simulink model "graph2"  (R2019a)
settings: Solver=VariableStepAuto  StartTime=0.0  StopTime=10.0  RelTol=1e-3
undefined symbols (not defined in the file or in its folder): av_simple, car, car_acc, genericAgentLib, LargeScaleSimLib_old, Objects, X, Y
libraries: robotlib x28, simulink x2
settings Model: Creator=agc3  LastModifiedBy=agc3

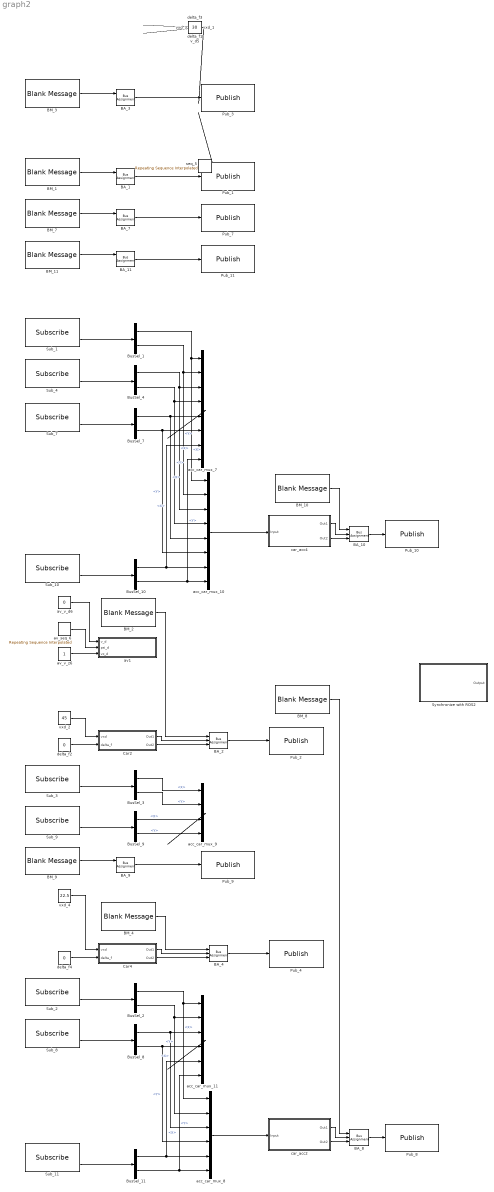
== system graph2 ==
  BA_{1..4,7..11} (9 alike) : BusAssignment  AssignedSignals=X,Y
  BM_{1..4,7..11} (9 alike) : robotlib/Blank Message  messageClass=Message  entityType=geometry_msgs/Point  messageType=geometry_msgs/Point  SampleTime=inf
      settings: SourceProductBaseCode=RO
  BusSel_{1..4,7..11} (9 alike) : BusSelector  OutputSignals=X,Y
  Car2 : Subsystem  AncestorBlock=LargeScaleSimLib_old/car  mask{obj=Objects{2}}
      mask prompts: obj "object"
      mask init:
      | set_param([gcb,'/ToWS'],'VariableName',obj.NameStrh)
  Car4 : Subsystem  AncestorBlock=LargeScaleSimLib_old/car  mask{obj=Objects{4}}
      mask prompts: obj "object"
      mask init:
      | set_param([gcb,'/ToWS'],'VariableName',obj.NameStrh)
  Pub_1 : robotlib/Publish  topicSource=Select from ROS network  topic=/Data_Pub_1  messageType=geometry_msgs/Point  messageQueueLength=1
      settings: SourceProductBaseCode=RO
  Pub_10 : robotlib/Publish  topicSource=Select from ROS network  topic=/Data_Pub_10  messageType=geometry_msgs/Point  messageQueueLength=1
      settings: SourceProductBaseCode=RO
  Pub_11 : robotlib/Publish  topicSource=Select from ROS network  topic=/Data_Pub_11  messageType=geometry_msgs/Point  messageQueueLength=1
      settings: SourceProductBaseCode=RO
  Pub_2 : robotlib/Publish  topicSource=Select from ROS network  topic=/Data_Pub_2  messageType=geometry_msgs/Point  messageQueueLength=1
      settings: SourceProductBaseCode=RO
  Pub_3 : robotlib/Publish  topicSource=Select from ROS network  topic=/Data_Pub_3  messageType=geometry_msgs/Point  messageQueueLength=1
      settings: SourceProductBaseCode=RO
  Pub_4 : robotlib/Publish  topicSource=Select from ROS network  topic=/Data_Pub_4  messageType=geometry_msgs/Point  messageQueueLength=1
      settings: SourceProductBaseCode=RO
  Pub_7 : robotlib/Publish  topicSource=Select from ROS network  topic=/Data_Pub_7  messageType=geometry_msgs/Point  messageQueueLength=1
      settings: SourceProductBaseCode=RO
  Pub_8 : robotlib/Publish  topicSource=Select from ROS network  topic=/Data_Pub_8  messageType=geometry_msgs/Point  messageQueueLength=1
      settings: SourceProductBaseCode=RO
  Pub_9 : robotlib/Publish  topicSource=Select from ROS network  topic=/Data_Pub_9  messageType=geometry_msgs/Point  messageQueueLength=1
      settings: SourceProductBaseCode=RO
  Sub_1 : robotlib/Subscribe  topicSource=Select from ROS network  topic=/Data_Pub_1  messageType=geometry_msgs/Point  sampleTime=-1  messageQueueLength=1
      settings: SourceProductBaseCode=RO
  Sub_10 : robotlib/Subscribe  topicSource=Select from ROS network  topic=/Data_Pub_10  messageType=geometry_msgs/Point  sampleTime=-1  messageQueueLength=1
      settings: SourceProductBaseCode=RO
  Sub_11 : robotlib/Subscribe  topicSource=Select from ROS network  topic=/Data_Pub_11  messageType=geometry_msgs/Point  sampleTime=-1  messageQueueLength=1
      settings: SourceProductBaseCode=RO
  Sub_2 : robotlib/Subscribe  topicSource=Select from ROS network  topic=/Data_Pub_2  messageType=geometry_msgs/Point  sampleTime=-1  messageQueueLength=1
      settings: SourceProductBaseCode=RO
  Sub_3 : robotlib/Subscribe  topicSource=Select from ROS network  topic=/Data_Pub_3  messageType=geometry_msgs/Point  sampleTime=-1  messageQueueLength=1
      settings: SourceProductBaseCode=RO
  Sub_4 : robotlib/Subscribe  topicSource=Select from ROS network  topic=/Data_Pub_4  messageType=geometry_msgs/Point  sampleTime=-1  messageQueueLength=1
      settings: SourceProductBaseCode=RO
  Sub_7 : robotlib/Subscribe  topicSource=Select from ROS network  topic=/Data_Pub_7  messageType=geometry_msgs/Point  sampleTime=-1  messageQueueLength=1
      settings: SourceProductBaseCode=RO
  Sub_8 : robotlib/Subscribe  topicSource=Select from ROS network  topic=/Data_Pub_8  messageType=geometry_msgs/Point  sampleTime=-1  messageQueueLength=1
      settings: SourceProductBaseCode=RO
  Sub_9 : robotlib/Subscribe  topicSource=Select from ROS network  topic=/Data_Pub_9  messageType=geometry_msgs/Point  sampleTime=-1  messageQueueLength=1
      settings: SourceProductBaseCode=RO
  Synchronize with ROS2 : Subsystem  Priority=1  TreatAsAtomicUnit=on
  acc_car_mux_10 : Mux  Inputs=8
  acc_car_mux_11 : Mux  Inputs=6
  acc_car_mux_7 : Mux  Inputs=8
  acc_car_mux_8 : Mux  Inputs=6
  acc_car_mux_9 : Mux
  av1 : Subsystem  AncestorBlock=genericAgentLib/av_simple  mask{obj=Objects{6}}
      mask prompts: obj "object"
      mask init:
      | set_param([gcb,'/ToWS'],'VariableName',obj.NameStrh)
  av_seq_6 : simulink/Sources/Repeating Sequence Interpolated  OutValues=[3 1 4 2 1].'  TimeValues=[0 0.1 0.5 0.6 1].'  LookUpMeth=Interpolation-Use End Values  tsamp=-1  OutMin=[]  OutMax=[]  OutDataTypeStr=double  OutputDataTypeScalingMode=double  OutDataType=fixdt(0,8)  OutScaling=2^-10
  av_v_d6 : Constant  Value=0
  av_v_z6 : Constant
  car_acc2 : Subsystem  AncestorBlock=LargeScaleSimLib_old/car_acc  mask{obj=Objects{8}}
      mask prompts: obj "object"
  car_acc4 : Subsystem  AncestorBlock=LargeScaleSimLib_old/car_acc  mask{obj=Objects{10}}
      mask prompts: obj "object"
  delta_f{1..4} (4 alike) : Constant  Value=0
  seq_5 : simulink/Sources/Repeating Sequence Interpolated  OutValues=[3 1 4 2 1].'  TimeValues=[0 0.1 0.5 0.6 1].'  LookUpMeth=Interpolation-Use End Values  tsamp=-1  OutMin=[]  OutMax=[]  OutDataTypeStr=double  OutputDataTypeScalingMode=double  OutDataType=fixdt(0,8)  OutScaling=2^-10
  v_d5 : Constant  Value=7.4003
  vxd_1 : Constant  Value=90
  vxd_2 : Constant  Value=45
  vxd_3 : Constant  Value=30
  vxd_4 : Constant  Value=22.5
  wires:
  ? -> BA_1/2
  ? -> BA_1/3
  vxd_1/1 -> ?
  delta_f1/1 -> ?
  ? -> BA_3/2
  ? -> BA_3/3
  vxd_3/1 -> ?
  delta_f3/1 -> ?
  v_d5/1 -> ?
  seq_5/1 -> ?
  ? -> BA_7/2
  ? -> BA_7/3
  acc_car_mux_7/1 -> ?
  ? -> BA_9/2
  ? -> BA_9/3
  acc_car_mux_9/1 -> ?
  ? -> BA_11/2
  ? -> BA_11/3
  acc_car_mux_11/1 -> ?
  BusSel_1/1 -> acc_car_mux_7/1, acc_car_mux_10/1  "<X>"
  BusSel_4/1 -> acc_car_mux_7/3, acc_car_mux_10/3  "<X>"
  BusSel_7/1 -> acc_car_mux_7/5, acc_car_mux_10/5  "<X>"
  BusSel_4/2 -> acc_car_mux_7/4, acc_car_mux_10/4  "<Y>"
  BusSel_10/2 -> acc_car_mux_7/8, acc_car_mux_10/8  "<Y>"
  BusSel_8/2 -> acc_car_mux_8/4, acc_car_mux_11/4  "<Y>"
  BusSel_11/2 -> acc_car_mux_8/6, acc_car_mux_11/6  "<Y>"
  BA_1/1 -> Pub_1/1
  BM_10/1 -> BA_10/1
  BusSel_10/1 -> acc_car_mux_7/7, acc_car_mux_10/7  "<X>"
  car_acc4/1(Out1) -> BA_10/2
  Car4/2(Out2) -> BA_4/3
  BusSel_9/1 -> acc_car_mux_9/3  "<X>"
  BM_2/1 -> BA_2/1
  car_acc4/2(Out2) -> BA_10/3
  BM_9/1 -> BA_9/1
  BA_10/1 -> Pub_10/1
  BM_11/1 -> BA_11/1
  Sub_8/2 -> BusSel_8/1
  Sub_3/2 -> BusSel_3/1
  BA_8/1 -> Pub_8/1
  BusSel_8/1 -> acc_car_mux_8/3, acc_car_mux_11/3  "<X>"
  Car4/1(Out1) -> BA_4/2
  BA_11/1 -> Pub_11/1
  BusSel_2/1 -> acc_car_mux_8/1, acc_car_mux_11/1  "<X>"
  BA_2/1 -> Pub_2/1
  BusSel_7/2 -> acc_car_mux_7/6, acc_car_mux_10/6  "<Y>"
  BusSel_3/1 -> acc_car_mux_9/1  "<X>"
  acc_car_mux_10/1 -> car_acc4/1(Input)
  BusSel_11/1 -> acc_car_mux_8/5, acc_car_mux_11/5  "<X>"
  BM_7/1 -> BA_7/1
  Sub_9/2 -> BusSel_9/1
  BusSel_3/2 -> acc_car_mux_9/2  "<Y>"
  acc_car_mux_8/1 -> car_acc2/1(Input)
  car_acc2/2(Out2) -> BA_8/3
  BM_8/1 -> BA_8/1
  BusSel_9/2 -> acc_car_mux_9/4  "<Y>"
  Sub_7/2 -> BusSel_7/1
  Car2/1(Out1) -> BA_2/2
  Sub_10/2 -> BusSel_10/1
  BusSel_2/2 -> acc_car_mux_8/2, acc_car_mux_11/2  "<Y>"
  Sub_4/2 -> BusSel_4/1
  Sub_1/2 -> BusSel_1/1
  car_acc2/1(Out1) -> BA_8/2
  BA_7/1 -> Pub_7/1
  Car2/2(Out2) -> BA_2/3
  delta_f4/1 -> Car4/2(delta_f)
  av_seq_6/1 -> av1/2(psi_d)
  av_v_d6/1 -> av1/1(v_d)
  Sub_11/2 -> BusSel_11/1
  vxd_4/1 -> Car4/1("vxd ")
  BM_1/1 -> BA_1/1
  vxd_2/1 -> Car2/1("vxd ")
  BA_9/1 -> Pub_9/1
  BA_4/1 -> Pub_4/1
  BusSel_1/2 -> acc_car_mux_7/2, acc_car_mux_10/2  "<Y>"
  BM_4/1 -> BA_4/1
  Sub_2/2 -> BusSel_2/1
  BA_3/1 -> Pub_3/1
  av_v_z6/1 -> av1/3(vz_d)
  BM_3/1 -> BA_3/1
  delta_f2/1 -> Car2/2(delta_f)

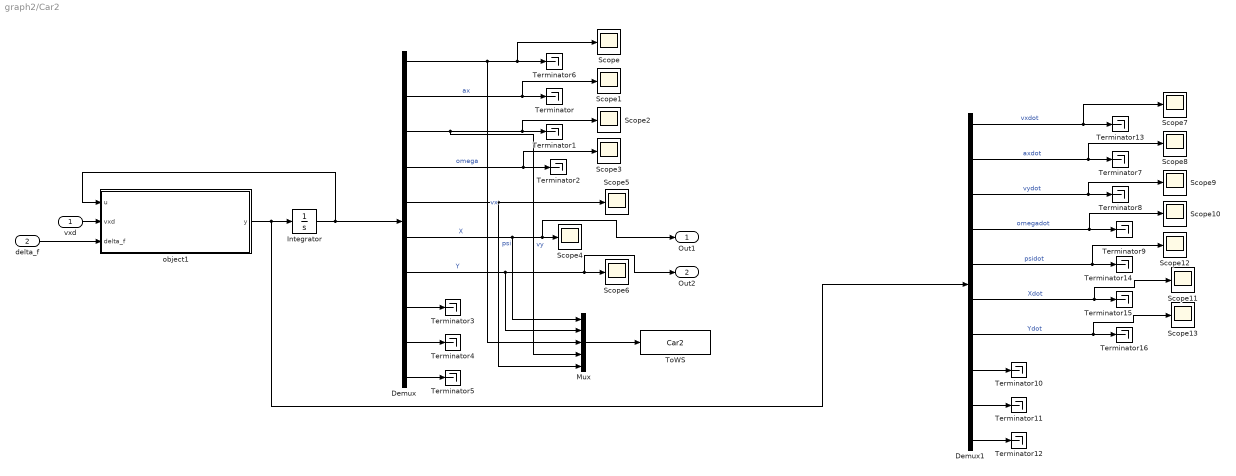
== system graph2/Car2 ==
  "vxd " : Inport
  delta_f : Inport  Port=2
  Demux : Demux  Outputs=10
  Demux1 : Demux  Outputs=10
  Integrator : Integrator  InitialCondition=obj.init
  Mux : Mux  Inputs=5
  Scope{,1..13} (14 alike) : Scope
  Terminator{,1..16} (17 alike) : Terminator
  ToWS : ToWorkspace  VariableName=Car2  SaveFormat=Timeseries  SampleTime=-1
  object1 : MATLAB Function  TreatAsAtomicUnit=on
  Out1 : Outport  VectorParamsAs1DForOutWhenUnconnected=on
  Out2 : Outport  Port=2  VectorParamsAs1DForOutWhenUnconnected=on
  wires:
  "vxd "/1 -> object1/2(vxd)
  Mux/1 -> ToWS/1
  object1/1(y) -> Integrator/1, Demux1/1
  Demux1/1 -> Scope7/1, Terminator13/1  "vxdot"
  Demux1/2 -> Scope8/1, Terminator7/1  "axdot"
  Demux1/3 -> Scope9/1, Terminator8/1  "vydot"
  Demux1/4 -> Scope10/1, Terminator9/1  "omegadot"
  Demux1/5 -> Scope12/1, Terminator14/1  "psidot"
  Demux1/6 -> Scope11/1, Terminator15/1  "Xdot"
  Demux1/7 -> Scope13/1, Terminator16/1  "Ydot"
  Demux1/8 -> Terminator10/1
  Demux1/9 -> Terminator11/1
  Demux1/10 -> Terminator12/1
  Demux/10 -> Terminator5/1
  Demux/9 -> Terminator4/1
  Demux/8 -> Terminator3/1
  Demux/7 -> Scope6/1, Out2/1, Mux/2  "Y"
  Demux/6 -> Scope4/1, Out1/1, Mux/1  "X"
  Demux/5 -> Scope5/1, Mux/5  "psi"
  Demux/4 -> Terminator2/1, Scope3/1  "omega"
  Demux/3 -> Terminator1/1, Scope2/1, Mux/4  "vy"
  Demux/2 -> Terminator/1, Scope1/1  "ax"
  Demux/1 -> Terminator6/1, Scope/1, Mux/3  "vx"
  delta_f/1 -> object1/3(delta_f)
  Integrator/1 -> object1/1(u), Demux/1

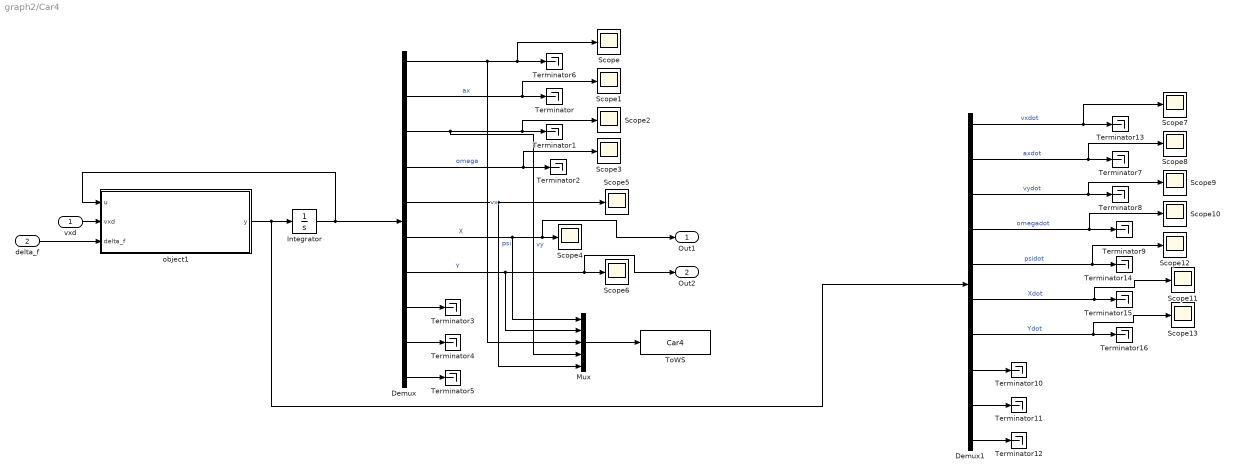
== system graph2/Car4 ==
  "vxd " : Inport
  delta_f : Inport  Port=2
  Demux : Demux  Outputs=10
  Demux1 : Demux  Outputs=10
  Integrator : Integrator  InitialCondition=obj.init
  Mux : Mux  Inputs=5
  Scope{,1..13} (14 alike) : Scope
  Terminator{,1..16} (17 alike) : Terminator
  ToWS : ToWorkspace  VariableName=Car4  SaveFormat=Timeseries  SampleTime=-1
  object1 : MATLAB Function  TreatAsAtomicUnit=on
  Out1 : Outport  VectorParamsAs1DForOutWhenUnconnected=on
  Out2 : Outport  Port=2  VectorParamsAs1DForOutWhenUnconnected=on
  wires:
  "vxd "/1 -> object1/2(vxd)
  Mux/1 -> ToWS/1
  object1/1(y) -> Integrator/1, Demux1/1
  Demux1/1 -> Scope7/1, Terminator13/1  "vxdot"
  Demux1/2 -> Scope8/1, Terminator7/1  "axdot"
  Demux1/3 -> Scope9/1, Terminator8/1  "vydot"
  Demux1/4 -> Scope10/1, Terminator9/1  "omegadot"
  Demux1/5 -> Scope12/1, Terminator14/1  "psidot"
  Demux1/6 -> Scope11/1, Terminator15/1  "Xdot"
  Demux1/7 -> Scope13/1, Terminator16/1  "Ydot"
  Demux1/8 -> Terminator10/1
  Demux1/9 -> Terminator11/1
  Demux1/10 -> Terminator12/1
  Demux/10 -> Terminator5/1
  Demux/9 -> Terminator4/1
  Demux/8 -> Terminator3/1
  Demux/7 -> Scope6/1, Out2/1, Mux/2  "Y"
  Demux/6 -> Scope4/1, Out1/1, Mux/1  "X"
  Demux/5 -> Scope5/1, Mux/5  "psi"
  Demux/4 -> Terminator2/1, Scope3/1  "omega"
  Demux/3 -> Terminator1/1, Scope2/1, Mux/4  "vy"
  Demux/2 -> Terminator/1, Scope1/1  "ax"
  Demux/1 -> Terminator6/1, Scope/1, Mux/3  "vx"
  delta_f/1 -> object1/3(delta_f)
  Integrator/1 -> object1/1(u), Demux/1

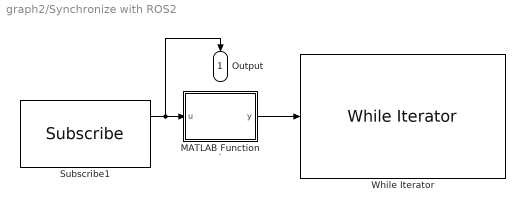
== system graph2/Synchronize with ROS2 ==
  note: `
  MATLAB Function : MATLAB Function  TreatAsAtomicUnit=on
  Subscribe1 : robotlib/Subscribe  topicSource=Select from ROS network  topic=/ClockTick  messageType=std_msgs/Float64  sampleTime=-1  messageQueueLength=1
      settings: SourceProductBaseCode=RO
  While Iterator : WhileIterator  MaxIters=-1  WhileBlockType=do-while  ShowIterationPort=on
  Output : Outport
  wires:
  Subscribe1/1 -> Output/1, MATLAB Function/1(u)
  MATLAB Function/1(y) -> While Iterator/1

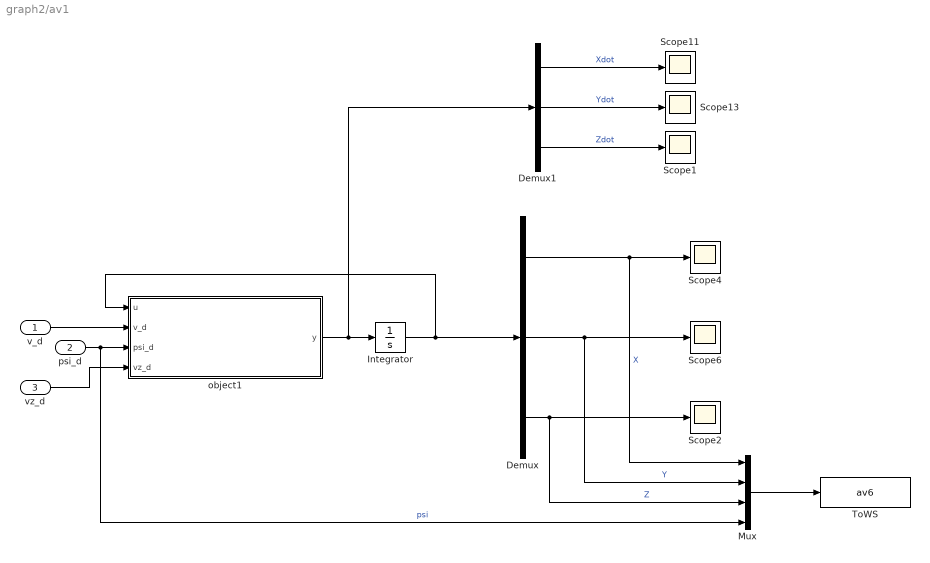
== system graph2/av1 ==
  v_d : Inport
  psi_d : Inport  Port=2
  vz_d : Inport  Port=3
  Demux : Demux  Outputs=3
  Demux1 : Demux  Outputs=3
  Integrator : Integrator  InitialCondition=obj.init
  Mux : Mux
  Scope{1..2,4,6,11,13} (6 alike) : Scope
  ToWS : ToWorkspace  VariableName=av6  SaveFormat=Timeseries  SampleTime=-1
  object1 : MATLAB Function  TreatAsAtomicUnit=on
  wires:
  Demux/2 -> Mux/2, Scope6/1  "Y"
  Demux/1 -> Mux/1, Scope4/1  "X"
  psi_d/1 -> Mux/4, object1/3(psi_d)  "psi"
  v_d/1 -> object1/2(v_d)
  Mux/1 -> ToWS/1
  object1/1(y) -> Integrator/1, Demux1/1
  Demux1/1 -> Scope11/1  "Xdot"
  Demux1/2 -> Scope13/1  "Ydot"
  Integrator/1 -> object1/1(u), Demux/1
  vz_d/1 -> object1/4(vz_d)
  Demux1/3 -> Scope1/1  "Zdot"
  Demux/3 -> Mux/3, Scope2/1  "Z"

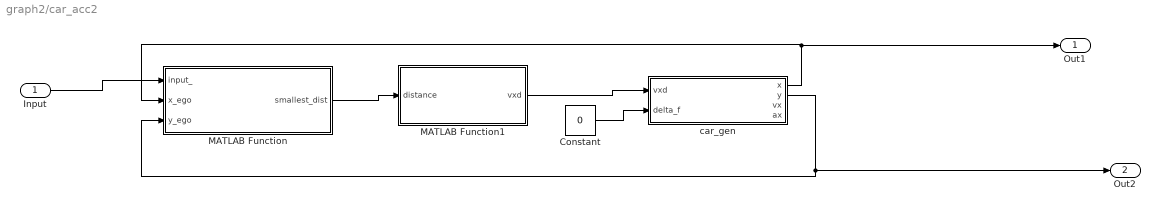
== system graph2/car_acc2 ==
  Input : Inport
  Constant : Constant  Value=0
  MATLAB Function : MATLAB Function  TreatAsAtomicUnit=on
  MATLAB Function1 : MATLAB Function  TreatAsAtomicUnit=on
  car_gen : Subsystem  AncestorBlock=genericAgentLib/car  mask{obj=obj}
      mask prompts: obj "object"
      mask init:
      | set_param([gcb,'/ToWS'],'VariableName',obj.NameStrh)
  Out1 : Outport  VectorParamsAs1DForOutWhenUnconnected=on
  Out2 : Outport  Port=2  VectorParamsAs1DForOutWhenUnconnected=on
  wires:
  MATLAB Function1/1(vxd) -> car_gen/1("vxd ")
  Constant/1 -> car_gen/2(delta_f)
  MATLAB Function/1(smallest_dist) -> MATLAB Function1/1(distance)
  Input/1 -> MATLAB Function/1(input_)
  car_gen/2(y) -> MATLAB Function/3(y_ego), Out2/1
  car_gen/1(x) -> MATLAB Function/2(x_ego), Out1/1

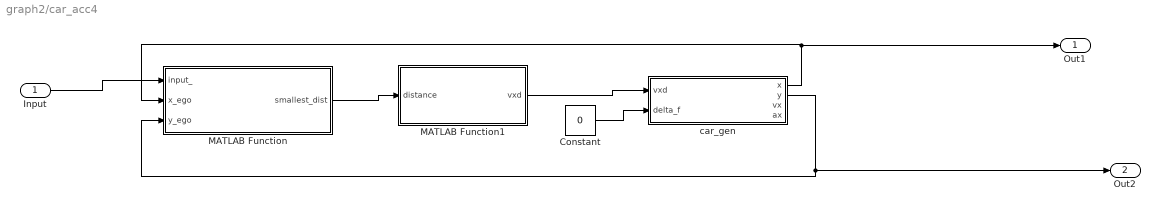
== system graph2/car_acc4 ==
  Input : Inport
  Constant : Constant  Value=0
  MATLAB Function : MATLAB Function  TreatAsAtomicUnit=on
  MATLAB Function1 : MATLAB Function  TreatAsAtomicUnit=on
  car_gen : Subsystem  AncestorBlock=genericAgentLib/car  mask{obj=obj}
      mask prompts: obj "object"
      mask init:
      | set_param([gcb,'/ToWS'],'VariableName',obj.NameStrh)
  Out1 : Outport  VectorParamsAs1DForOutWhenUnconnected=on
  Out2 : Outport  Port=2  VectorParamsAs1DForOutWhenUnconnected=on
  wires:
  MATLAB Function1/1(vxd) -> car_gen/1("vxd ")
  Constant/1 -> car_gen/2(delta_f)
  MATLAB Function/1(smallest_dist) -> MATLAB Function1/1(distance)
  Input/1 -> MATLAB Function/1(input_)
  car_gen/2(y) -> MATLAB Function/3(y_ego), Out2/1
  car_gen/1(x) -> MATLAB Function/2(x_ego), Out1/1

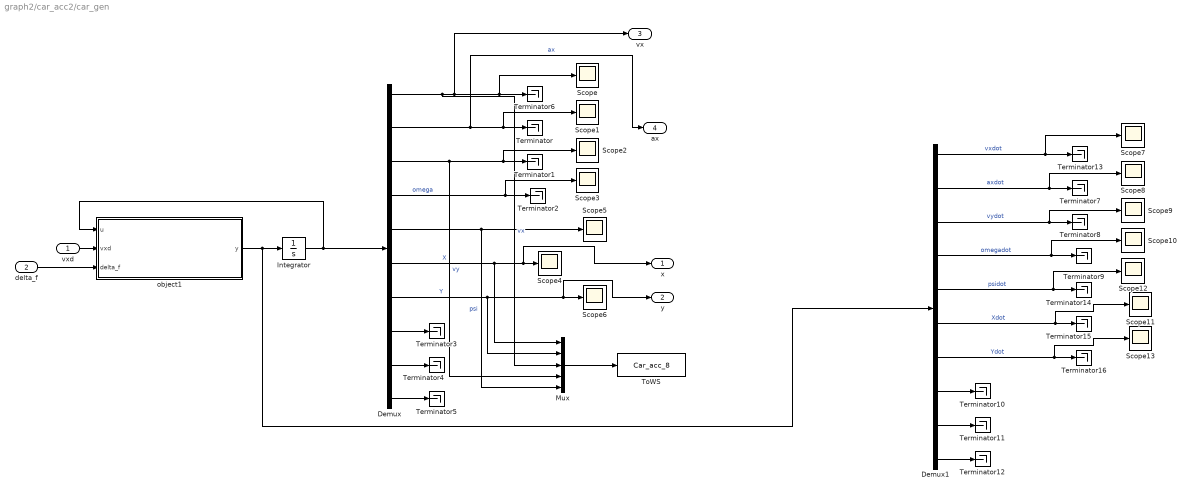
== system graph2/car_acc2/car_gen ==
  "vxd " : Inport
  delta_f : Inport  Port=2
  Demux : Demux  Outputs=10
  Demux1 : Demux  Outputs=10
  Integrator : Integrator  InitialCondition=obj.init
  Mux : Mux  Inputs=5
  Scope{,1..13} (14 alike) : Scope
  Terminator{,1..16} (17 alike) : Terminator
  ToWS : ToWorkspace  VariableName=Car_acc_8  SaveFormat=Timeseries  SampleTime=-1
  object1 : MATLAB Function  TreatAsAtomicUnit=on
  x : Outport  VectorParamsAs1DForOutWhenUnconnected=on
  y : Outport  Port=2  VectorParamsAs1DForOutWhenUnconnected=on
  vx : Outport  Port=3  VectorParamsAs1DForOutWhenUnconnected=on
  "ax " : Outport  Port=4  VectorParamsAs1DForOutWhenUnconnected=on
  wires:
  "vxd "/1 -> object1/2(vxd)
  Mux/1 -> ToWS/1
  object1/1(y) -> Integrator/1, Demux1/1
  Demux1/1 -> Scope7/1, Terminator13/1  "vxdot"
  Demux1/2 -> Scope8/1, Terminator7/1  "axdot"
  Demux1/3 -> Scope9/1, Terminator8/1  "vydot"
  Demux1/4 -> Scope10/1, Terminator9/1  "omegadot"
  Demux1/5 -> Scope12/1, Terminator14/1  "psidot"
  Demux1/6 -> Scope11/1, Terminator15/1  "Xdot"
  Demux1/7 -> Scope13/1, Terminator16/1  "Ydot"
  Demux1/8 -> Terminator10/1
  Demux1/9 -> Terminator11/1
  Demux1/10 -> Terminator12/1
  Demux/10 -> Terminator5/1
  Demux/9 -> Terminator4/1
  Demux/8 -> Terminator3/1
  Demux/7 -> Scope6/1, y/1, Mux/2  "Y"
  Demux/6 -> Scope4/1, x/1, Mux/1  "X"
  Demux/5 -> Scope5/1, Mux/5  "psi"
  Demux/4 -> Terminator2/1, Scope3/1  "omega"
  Demux/3 -> Terminator1/1, Scope2/1, Mux/4  "vy"
  Demux/2 -> Terminator/1, Scope1/1, "ax "/1  "ax"
  Demux/1 -> Terminator6/1, Scope/1, vx/1, Mux/3  "vx"
  delta_f/1 -> object1/3(delta_f)
  Integrator/1 -> object1/1(u), Demux/1

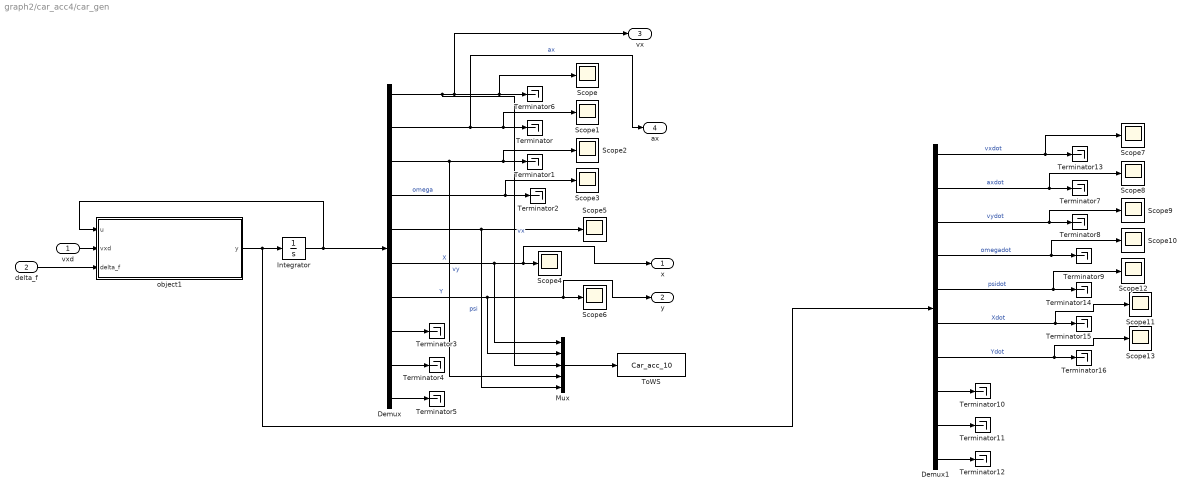
== system graph2/car_acc4/car_gen ==
  "vxd " : Inport
  delta_f : Inport  Port=2
  Demux : Demux  Outputs=10
  Demux1 : Demux  Outputs=10
  Integrator : Integrator  InitialCondition=obj.init
  Mux : Mux  Inputs=5
  Scope{,1..13} (14 alike) : Scope
  Terminator{,1..16} (17 alike) : Terminator
  ToWS : ToWorkspace  VariableName=Car_acc_10  SaveFormat=Timeseries  SampleTime=-1
  object1 : MATLAB Function  TreatAsAtomicUnit=on
  x : Outport  VectorParamsAs1DForOutWhenUnconnected=on
  y : Outport  Port=2  VectorParamsAs1DForOutWhenUnconnected=on
  vx : Outport  Port=3  VectorParamsAs1DForOutWhenUnconnected=on
  "ax " : Outport  Port=4  VectorParamsAs1DForOutWhenUnconnected=on
  wires:
  "vxd "/1 -> object1/2(vxd)
  Mux/1 -> ToWS/1
  object1/1(y) -> Integrator/1, Demux1/1
  Demux1/1 -> Scope7/1, Terminator13/1  "vxdot"
  Demux1/2 -> Scope8/1, Terminator7/1  "axdot"
  Demux1/3 -> Scope9/1, Terminator8/1  "vydot"
  Demux1/4 -> Scope10/1, Terminator9/1  "omegadot"
  Demux1/5 -> Scope12/1, Terminator14/1  "psidot"
  Demux1/6 -> Scope11/1, Terminator15/1  "Xdot"
  Demux1/7 -> Scope13/1, Terminator16/1  "Ydot"
  Demux1/8 -> Terminator10/1
  Demux1/9 -> Terminator11/1
  Demux1/10 -> Terminator12/1
  Demux/10 -> Terminator5/1
  Demux/9 -> Terminator4/1
  Demux/8 -> Terminator3/1
  Demux/7 -> Scope6/1, y/1, Mux/2  "Y"
  Demux/6 -> Scope4/1, x/1, Mux/1  "X"
  Demux/5 -> Scope5/1, Mux/5  "psi"
  Demux/4 -> Terminator2/1, Scope3/1  "omega"
  Demux/3 -> Terminator1/1, Scope2/1, Mux/4  "vy"
  Demux/2 -> Terminator/1, Scope1/1, "ax "/1  "ax"
  Demux/1 -> Terminator6/1, Scope/1, vx/1, Mux/3  "vx"
  delta_f/1 -> object1/3(delta_f)
  Integrator/1 -> object1/1(u), Demux/1

== matlab function graph2/Car2/object1 ==
  data: u input size=10; vxd input size=1; delta_f input size=1; y output size=10; obj parameter
function y = fcn(u,vxd, delta_f, obj)

vx = u(1);
ax = u(2);
vy = u(3);
omega = u(4);
psi = u(5);
X = u(6);
Y = u(7);

if abs(vx)> obj.vx_threshold1
    alpha_f = delta_f * pi/180 - (vy + omega * obj.lf) / vx;
    alpha_r = - (vy - omega * obj.lr) / vx;
else
    alpha_f = 0;
    alpha_r = 0;
end

Fx = obj.m * ax;
Fyf = min(obj.Fyfmax,obj.Calpha_f * alpha_f);
Fyr = min(obj.Fyrmax, obj.Calpha_r * alpha_r);
Fy = Fyf + Fyr;

M  = Fyf * obj.lf - Fyr * obj.lr;

omegadot = M / obj.I;
%        vxdot = Fx / obj.m + omega * vy;
vxdot = ax;
axdot = - 2 * obj.longctl.psi * obj.longctl.w* ax - (obj.longctl.w)^2 * (vx - vxd);
vydot = Fy / obj.m - omega * vx;
psidot = omega;
t1 = TF(psi) * [vx;vy];
Xdot = t1(1);
Ydot = t1(2);
y = [vxdot, axdot, vydot, omegadot, psidot, Xdot, Ydot, 0 0 0]';
end

function y = TF(psi)
y = [cos(psi), sin(psi); -sin(psi), cos(psi)];
end

== matlab function graph2/Car4/object1 ==
  data: u input size=10; vxd input size=1; delta_f input size=1; y output size=10; obj parameter
function y = fcn(u,vxd, delta_f, obj)

vx = u(1);
ax = u(2);
vy = u(3);
omega = u(4);
psi = u(5);
X = u(6);
Y = u(7);

if abs(vx)> obj.vx_threshold1
    alpha_f = delta_f * pi/180 - (vy + omega * obj.lf) / vx;
    alpha_r = - (vy - omega * obj.lr) / vx;
else
    alpha_f = 0;
    alpha_r = 0;
end

Fx = obj.m * ax;
Fyf = min(obj.Fyfmax,obj.Calpha_f * alpha_f);
Fyr = min(obj.Fyrmax, obj.Calpha_r * alpha_r);
Fy = Fyf + Fyr;

M  = Fyf * obj.lf - Fyr * obj.lr;

omegadot = M / obj.I;
%        vxdot = Fx / obj.m + omega * vy;
vxdot = ax;
axdot = - 2 * obj.longctl.psi * obj.longctl.w* ax - (obj.longctl.w)^2 * (vx - vxd);
vydot = Fy / obj.m - omega * vx;
psidot = omega;
t1 = TF(psi) * [vx;vy];
Xdot = t1(1);
Ydot = t1(2);
y = [vxdot, axdot, vydot, omegadot, psidot, Xdot, Ydot, 0 0 0]';
end

function y = TF(psi)
y = [cos(psi), sin(psi); -sin(psi), cos(psi)];
end

== matlab function graph2/Synchronize with ROS2/MATLAB Function ==
  data: u input; y output
function y = fcn_graph1(u)

%pause(0.001);
persistent flag;

if isempty(flag)
   flag = 0; 
end

if(u == 1)
    
    if (flag == 0)
       y = 0;
       flag = 1;
       
    elseif(flag == 1)
        y = 0;
       
    else
        y = 1;
        
    end
else
    pause(0.001);
    if(flag == 1)
        y = 0;
    else
        y=1;
    end
end

== matlab function graph2/av1/object1 ==
  data: u input; v_d input; psi_d input; vz_d input; y output size=3; obj parameter
function y = fcn(u, v_d, psi_d, vz_d, obj)

Z = u(3);
Xdot = v_d * cos(psi_d);
Ydot = v_d * sin(psi_d);
if Z <= 0 && vz_d < 0
   Zdot = 0;
else
   Zdot = vz_d;
end
y = [Xdot, Ydot, Zdot]';
end

function y = TF(psi)
y = [cos(psi), sin(psi); -sin(psi), cos(psi)];
end

== matlab function graph2/car_acc2/MATLAB Function ==
  data: input_ input; smallest_dist output; x_ego input; y_ego input
function smallest_dist = sensor(input_, x_ego, y_ego)

smallest_d = inf;
x = 1;


for c = 1:(length(input_)/2)

    temp_d = sqrt((x_ego - input_(x))^2+(y_ego-input_(x+1))^2);
    
    if ((smallest_d > temp_d) && (temp_d > 1) &&((input_(x) > x_ego)))% &&~(y_ego == input_(x+1)) )
        
        smallest_d = temp_d;
        
    end
    x = x+2;
    
end


smallest_dist = smallest_d;

== matlab function graph2/car_acc2/MATLAB Function1 ==
  data: vxd output; distance input
function vxd = fcn(distance)

d_thres1 = 80;
d_thres2 = 100;
vx_ref = 30;
kp = 0.001;
cc = 1;
vxd = 1;
if(cc)
    v_des = vx_ref;
    if(distance <= d_thres1)
        cc = 0;
    else
        cc = 1;%redunadnt statement
    end
else 
    v_des = vx_ref - kp*(d_thres1 - distance);
    if(distance > d_thres2)
        cc = 1;
    else
        cc = 0;%redundant statement
    end
end

% 
% if((distance <=  d_thres1))
%     v_des = vx_ref - kp*(d_thres1 - distance);
% elseif (distance > d_thres2)
%     v_des = vx_ref;
% else
%     v_des = vx_ref;
% end


vxd = v_des;

== matlab function graph2/car_acc2/car_gen/object1 ==
  data: u input size=10; vxd input size=1; delta_f input size=1; y output size=10; obj parameter
function y = fcn(u,vxd, delta_f, obj)

vx = u(1);
ax = u(2);
vy = u(3);
omega = u(4);
psi = u(5);
X = u(6);
Y = u(7);

if abs(vx)> obj.vx_threshold1
    alpha_f = delta_f * pi/180 - (vy + omega * obj.lf) / vx;
    alpha_r = - (vy - omega * obj.lr) / vx;
else
    alpha_f = 0;
    alpha_r = 0;
end

Fx = obj.m * ax;
Fyf = min(obj.Fyfmax,obj.Calpha_f * alpha_f);
Fyr = min(obj.Fyrmax, obj.Calpha_r * alpha_r);
Fy = Fyf + Fyr;

M  = Fyf * obj.lf - Fyr * obj.lr;

omegadot = M / obj.I;
%        vxdot = Fx / obj.m + omega * vy;
vxdot = ax;
axdot = - 2 * obj.longctl.psi * obj.longctl.w* ax - (obj.longctl.w)^2 * (vx - vxd);
vydot = Fy / obj.m - omega * vx;
psidot = omega;
t1 = TF(psi) * [vx;vy];
Xdot = t1(1);
Ydot = t1(2);
y = [vxdot, axdot, vydot, omegadot, psidot, Xdot, Ydot, 0 0 0]';
end

function y = TF(psi)
y = [cos(psi), sin(psi); -sin(psi), cos(psi)];
end

== matlab function graph2/car_acc4/MATLAB Function ==
  data: input_ input; smallest_dist output; x_ego input; y_ego input
function smallest_dist = sensor(input_, x_ego, y_ego)

smallest_d = inf;
x = 1;


for c = 1:(length(input_)/2)

    temp_d = sqrt((x_ego - input_(x))^2+(y_ego-input_(x+1))^2);
    
    if ((smallest_d > temp_d) && (temp_d > 1) &&((input_(x) > x_ego)))% &&~(y_ego == input_(x+1)) )
        
        smallest_d = temp_d;
        
    end
    x = x+2;
    
end


smallest_dist = smallest_d;

== matlab function graph2/car_acc4/MATLAB Function1 ==
  data: vxd output; distance input
function vxd = fcn(distance)

d_thres1 = 80;
d_thres2 = 100;
vx_ref = 30;
kp = 0.001;
cc = 1;
vxd = 1;
if(cc)
    v_des = vx_ref;
    if(distance <= d_thres1)
        cc = 0;
    else
        cc = 1;%redunadnt statement
    end
else 
    v_des = vx_ref - kp*(d_thres1 - distance);
    if(distance > d_thres2)
        cc = 1;
    else
        cc = 0;%redundant statement
    end
end

% 
% if((distance <=  d_thres1))
%     v_des = vx_ref - kp*(d_thres1 - distance);
% elseif (distance > d_thres2)
%     v_des = vx_ref;
% else
%     v_des = vx_ref;
% end


vxd = v_des;

== matlab function graph2/car_acc4/car_gen/object1 ==
  data: u input size=10; vxd input size=1; delta_f input size=1; y output size=10; obj parameter
function y = fcn(u,vxd, delta_f, obj)

vx = u(1);
ax = u(2);
vy = u(3);
omega = u(4);
psi = u(5);
X = u(6);
Y = u(7);

if abs(vx)> obj.vx_threshold1
    alpha_f = delta_f * pi/180 - (vy + omega * obj.lf) / vx;
    alpha_r = - (vy - omega * obj.lr) / vx;
else
    alpha_f = 0;
    alpha_r = 0;
end

Fx = obj.m * ax;
Fyf = min(obj.Fyfmax,obj.Calpha_f * alpha_f);
Fyr = min(obj.Fyrmax, obj.Calpha_r * alpha_r);
Fy = Fyf + Fyr;

M  = Fyf * obj.lf - Fyr * obj.lr;

omegadot = M / obj.I;
%        vxdot = Fx / obj.m + omega * vy;
vxdot = ax;
axdot = - 2 * obj.longctl.psi * obj.longctl.w* ax - (obj.longctl.w)^2 * (vx - vxd);
vydot = Fy / obj.m - omega * vx;
psidot = omega;
t1 = TF(psi) * [vx;vy];
Xdot = t1(1);
Ydot = t1(2);
y = [vxdot, axdot, vydot, omegadot, psidot, Xdot, Ydot, 0 0 0]';
end

function y = TF(psi)
y = [cos(psi), sin(psi); -sin(psi), cos(psi)];
end
